simulink model "LQ_point_1"  (R2021b)
settings: Solver=VariableStepAuto  StartTime=0.0  StopTime=10.0  RelTol=1e-3
values from neighbouring files (symbols this model uses):
  A = sysd.A    [main4.m]
  B = sysd.B    [main4.m]
  C = sysd.C    [main4.m]
  C_temp = eye(length(A))    [main4.m]
  D_temp = zeros(length(B), 1)    [main4.m]
  LQ_d_1 = dlqr(A, B, Q_LQ_1, R_LQ_1 )    [main4.m]
  LQ_d_2 = dlqr(A, B, Q_LQ_2, R_LQ_1 )    [main4.m]
  T_sampling = 0.1    [main4.m]
  u_max = 5    [main4.m]
  u_min = -5    [main4.m]
  x_0 = [0 10]'    [main4.m]
settings Model: Creator=PaoloA  LastModifiedBy=PaoloA

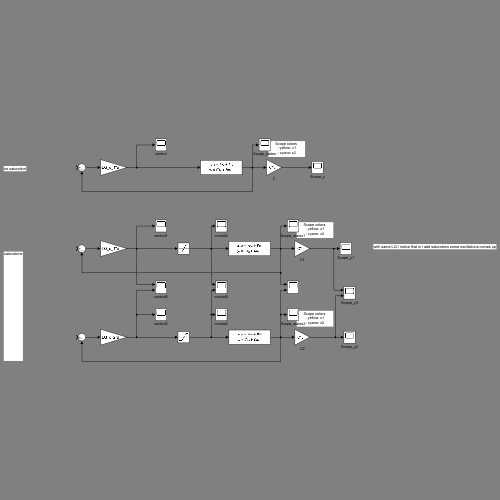
[thumbnail: Simulink's stored preview of the top-level diagram]
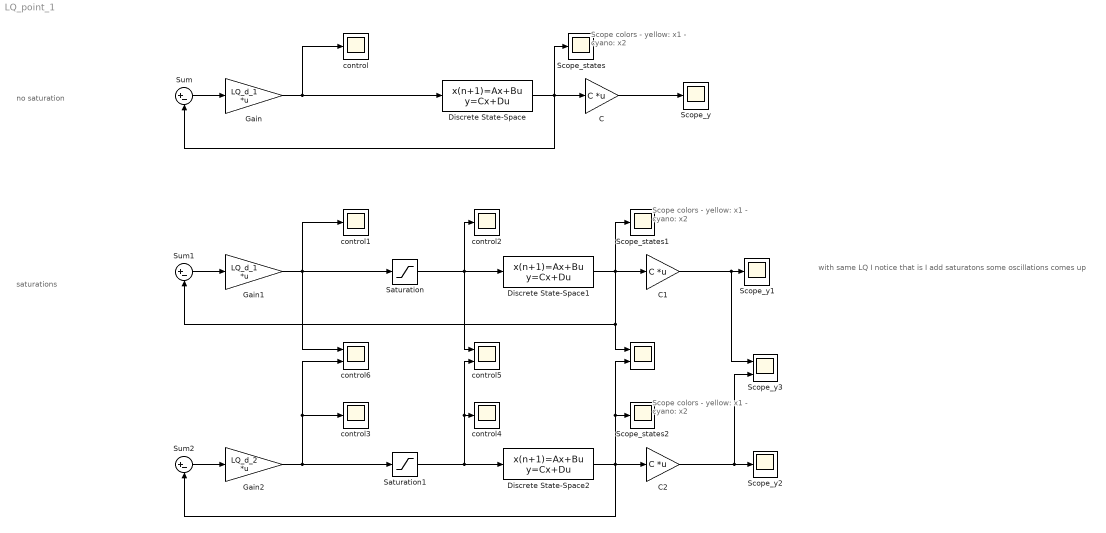
== system LQ_point_1 ==
  note: with same LQ I notice that is I add saturatons some oscillations comes up
  note: saturations
  note: no saturation
  note: Scope colors
      | - yellow: x1
      | - cyano: x2
  note: Scope colors
      | - yellow: x1
      | - cyano: x2
  note: Scope colors
      | - yellow: x1
      | - cyano: x2
  " " : Scope  NumInputPorts=2
  C : Gain  Gain=C  Multiplication=Matrix(K*u)
  C1 : Gain  Gain=C  Multiplication=Matrix(K*u)
  C2 : Gain  Gain=C  Multiplication=Matrix(K*u)
  Discrete State-Space : DiscreteStateSpace  A=A  B=B  C=C_temp  D=D_temp  InitialCondition=x_0  SampleTime=T_sampling
  Discrete State-Space1 : DiscreteStateSpace  A=A  B=B  C=C_temp  D=D_temp  InitialCondition=x_0  SampleTime=T_sampling
  Discrete State-Space2 : DiscreteStateSpace  A=A  B=B  C=C_temp  D=D_temp  InitialCondition=x_0  SampleTime=T_sampling
  Gain : Gain  Gain=LQ_d_1  Multiplication=Matrix(K*u)
  Gain1 : Gain  Gain=LQ_d_1  Multiplication=Matrix(K*u)
  Gain2 : Gain  Gain=LQ_d_2  Multiplication=Matrix(K*u)
  Saturation : Saturate  UpperLimit=u_max  LowerLimit=u_min
  Saturation1 : Saturate  UpperLimit=u_max  LowerLimit=u_min
  Scope_states : Scope
  Scope_states1 : Scope
  Scope_states2 : Scope
  Scope_y : Scope
  Scope_y1 : Scope
  Scope_y2 : Scope
  Scope_y3 : Scope  NumInputPorts=2
  Sum : Sum  Inputs=|+-
  Sum1 : Sum  Inputs=|+-
  Sum2 : Sum  Inputs=|+-
  control{,1..4} (5 alike) : Scope
  control5 : Scope  NumInputPorts=2
  control6 : Scope  NumInputPorts=2
  wires:
  Discrete State-Space/1 -> C/1, Scope_states/1, Sum/2
  C/1 -> Scope_y/1
  Sum/1 -> Gain/1
  Gain/1 -> Discrete State-Space/1, control/1
  Gain1/1 -> control6/1, Saturation/1, control1/1
  Sum1/1 -> Gain1/1
  C1/1 -> Scope_y3/1, Scope_y1/1
  Discrete State-Space1/1 -> C1/1, Scope_states1/1, " "/1, Sum1/2
  Saturation/1 -> control5/1, control2/1, Discrete State-Space1/1
  Discrete State-Space2/1 -> C2/1, " "/2, Scope_states2/1, Sum2/2
  C2/1 -> Scope_y3/2, Scope_y2/1
  Sum2/1 -> Gain2/1
  Gain2/1 -> Saturation1/1, control3/1, control6/2
  Saturation1/1 -> control5/2, control4/1, Discrete State-Space2/1
